simulink model "simulinkMonkey"  (R2019b)
settings: Solver=VariableStepAuto  StartTime=0.0  StopTime=3  RelTol=1e-3
values from neighbouring files (symbols this model uses):
  dq0_sim = T(1, 13:19)    [prepSimulink.m]
  q0_sim = T(1, 6:12)    [prepSimulink.m]
libraries: simulink x2
settings Model: Creator=Mike Dermksian  LastModifiedBy=Mike Dermksian

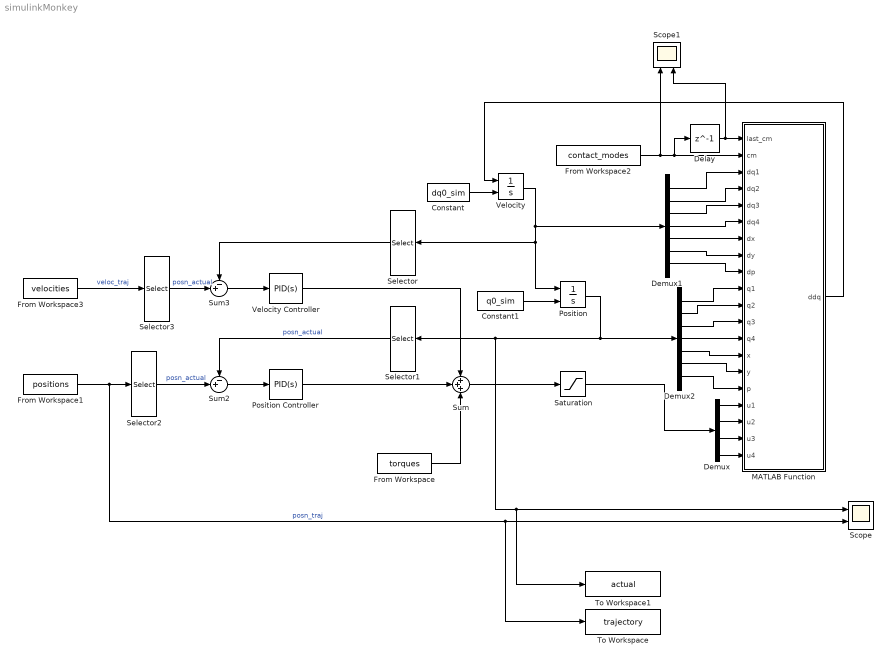
== system simulinkMonkey ==
  Constant : Constant  Value=dq0_sim
  Constant1 : Constant  Value=q0_sim
  Delay : Delay  DelayLength=1  InitialCondition=12
  Demux : Demux
  Demux1 : Demux  Outputs=7
  Demux2 : Demux  Outputs=7
  From Workspace : FromWorkspace  VariableName=torques  SampleTime=0  Interpolate=off  OutputAfterFinalValue=Setting to zero
  From Workspace1 : FromWorkspace  VariableName=positions  SampleTime=0  OutputAfterFinalValue=Holding final value
  From Workspace2 : FromWorkspace  VariableName=contact_modes  SampleTime=0  Interpolate=off  OutputAfterFinalValue=Holding final value
  From Workspace3 : FromWorkspace  VariableName=velocities  SampleTime=0  OutputAfterFinalValue=Holding final value
  MATLAB Function : MATLAB Function  TreatAsAtomicUnit=on
  Position : Integrator  InitialConditionSource=external
  Position Controller : simulink/Continuous/PID Controller  Controller=PID  Form=Parallel  TimeDomain=Continuous-time  SampleTime=-1  IntegratorMethod=Forward Euler  FilterMethod=Forward Euler  ControllerParametersSource=internal  P=100  I=10  D=0.1  UseFilter=on  N=100  TunerSelectOption=Transfer Function Based (PID Tuner App)  InitialConditionSource=internal  InitialConditionForIntegrator=0  InitialConditionForFilter=0  DifferentiatorICPrevScaledInput=0  ExternalReset=none  TrackingMode=off  Kt=1  LimitOutput=off  UpperSaturationLimit=inf  LowerSaturationLimit=-inf  LinearizeAsGain=on  AntiWindupMode=none  Kb=1  POutMin=[]  POutMax=[]  IOutMin=[]  IOutMax=[]  DOutMin=[]  DOutMax=[]  NOutMin=[]  NOutMax=[]  SumOutMin=[]  SumOutMax=[]  SaturationOutMin=[]  SaturationOutMax=[]  PParamMin=[]  PParamMax=[]  IParamMin=[]  IParamMax=[]  DParamMin=[]  DParamMax=[]  NParamMin=[]  NParamMax=[]  KbParamMin=[]  KbParamMax=[]  KtParamMin=[]  KtParamMax=[]  KbOutMin=[]  KbOutMax=[]  KtOutMin=[]  KtOutMax=[]  IntegratorOutMin=[]  IntegratorOutMax=[]  FilterOutMin=[]  FilterOutMax=[]  SumI1OutMin=[]  SumI1OutMax=[]  SumI2OutMin=[]  SumI2OutMax=[]  SumI3OutMin=[]  SumI3OutMax=[]  SumI4OutMin=[]  SumI4OutMax=[]  SumDOutMin=[]  SumDOutMax=[]  DifferentiatorOutMin=[]  DifferentiatorOutMax=[]  FilterDiffOutCoefMin=[]  FilterDiffOutCoefMax=[]  ReciprocalOutMin=[]  ReciprocalOutMax=[]  SumDenOutMin=[]  SumDenOutMax=[]  SumNumOutMin=[]  SumNumOutMax=[]  DivideOutMin=[]  DivideOutMax=[]  IntegratorContinuousStateAttributes=''  IntegratorStateMustResolveToSignalObject=off  IntegratorRTWStateStorageClass=Auto  FilterContinuousStateAttributes=''  FilterStateMustResolveToSignalObject=off  FilterRTWStateStorageClass=Auto  ParallelPVariant=InternalParameters  IdealPVariant=Disabled  IVariant=InternalParameters  DVariant=InternalParameters  IntegratorVariant=Continuous  SatVariant=Disabled  AWVariant=Passthrough  PCopyVariant=Disabled  TRVariant=Disabled  FdbkBlocksVariant=Forward  IdealPFdbkVariant=Disabled  SatFdbkVariant=Disabled  DerivativeFilterVariant=ContFilter  NVariant=InternalParameters  NCopyVariant=Disabled  FilterICVariant=InternalICsFilter  IntegratorICVariant=InternalICs  ExternalResetVariant=Disabled  TRSumVariant=Passthrough  SumFdbkVariant=Disabled  SumVariant=Sum_PID
  Saturation : Saturate  UpperLimit=3  LowerLimit=-3
  Scope : Scope  NumInputPorts=2
  Scope1 : Scope  NumInputPorts=2
  Selector{,1..3} (4 alike) : Selector  InputPortWidth=7  IndexOptions=Index vector (dialog)  Indices=[1 2 3 4]  OutputSizes=1
  Sum : Sum  Inputs=+++
  Sum2 : Sum  Inputs=-+|
  Sum3 : Sum  Inputs=-+|
  To Workspace : ToWorkspace  VariableName=trajectory  SampleTime=-1
  To Workspace1 : ToWorkspace  VariableName=actual  SampleTime=-1
  Velocity : Integrator  InitialConditionSource=external
  Velocity Controller : simulink/Continuous/PID Controller  Controller=PID  Form=Parallel  TimeDomain=Continuous-time  SampleTime=-1  IntegratorMethod=Forward Euler  FilterMethod=Forward Euler  ControllerParametersSource=internal  P=100  I=10  D=0.1  UseFilter=on  N=100  TunerSelectOption=Transfer Function Based (PID Tuner App)  InitialConditionSource=internal  InitialConditionForIntegrator=0  InitialConditionForFilter=0  DifferentiatorICPrevScaledInput=0  ExternalReset=none  TrackingMode=off  Kt=1  LimitOutput=off  UpperSaturationLimit=inf  LowerSaturationLimit=-inf  LinearizeAsGain=on  AntiWindupMode=none  Kb=1  POutMin=[]  POutMax=[]  IOutMin=[]  IOutMax=[]  DOutMin=[]  DOutMax=[]  NOutMin=[]  NOutMax=[]  SumOutMin=[]  SumOutMax=[]  SaturationOutMin=[]  SaturationOutMax=[]  PParamMin=[]  PParamMax=[]  IParamMin=[]  IParamMax=[]  DParamMin=[]  DParamMax=[]  NParamMin=[]  NParamMax=[]  KbParamMin=[]  KbParamMax=[]  KtParamMin=[]  KtParamMax=[]  KbOutMin=[]  KbOutMax=[]  KtOutMin=[]  KtOutMax=[]  IntegratorOutMin=[]  IntegratorOutMax=[]  FilterOutMin=[]  FilterOutMax=[]  SumI1OutMin=[]  SumI1OutMax=[]  SumI2OutMin=[]  SumI2OutMax=[]  SumI3OutMin=[]  SumI3OutMax=[]  SumI4OutMin=[]  SumI4OutMax=[]  SumDOutMin=[]  SumDOutMax=[]  DifferentiatorOutMin=[]  DifferentiatorOutMax=[]  FilterDiffOutCoefMin=[]  FilterDiffOutCoefMax=[]  ReciprocalOutMin=[]  ReciprocalOutMax=[]  SumDenOutMin=[]  SumDenOutMax=[]  SumNumOutMin=[]  SumNumOutMax=[]  DivideOutMin=[]  DivideOutMax=[]  IntegratorContinuousStateAttributes=''  IntegratorStateMustResolveToSignalObject=off  IntegratorRTWStateStorageClass=Auto  FilterContinuousStateAttributes=''  FilterStateMustResolveToSignalObject=off  FilterRTWStateStorageClass=Auto  ParallelPVariant=InternalParameters  IdealPVariant=Disabled  IVariant=InternalParameters  DVariant=InternalParameters  IntegratorVariant=Continuous  SatVariant=Disabled  AWVariant=Passthrough  PCopyVariant=Disabled  TRVariant=Disabled  FdbkBlocksVariant=Forward  IdealPFdbkVariant=Disabled  SatFdbkVariant=Disabled  DerivativeFilterVariant=ContFilter  NVariant=InternalParameters  NCopyVariant=Disabled  FilterICVariant=InternalICsFilter  IntegratorICVariant=InternalICs  ExternalResetVariant=Disabled  TRSumVariant=Passthrough  SumFdbkVariant=Disabled  SumVariant=Sum_PID
  wires:
  Velocity/1 -> Position/1, Selector/1, Demux1/1
  MATLAB Function/1(ddq) -> Velocity/1
  Position/1 -> Demux2/1, Scope/1, To Workspace1/1, Selector1/1
  Demux/1 -> MATLAB Function/17(u1)
  Demux/2 -> MATLAB Function/18(u2)
  Demux/3 -> MATLAB Function/19(u3)
  Demux/4 -> MATLAB Function/20(u4)
  Constant/1 -> Velocity/2
  Constant1/1 -> Position/2
  Sum/1 -> Saturation/1
  Sum2/1 -> Position Controller/1
  From Workspace1/1 -> To Workspace/1, Scope/2, Selector2/1  "posn_traj"
  From Workspace2/1 -> MATLAB Function/2(cm), Delay/1, Scope1/1
  Selector/1 -> Sum3/1
  Selector1/1 -> Sum2/1  "posn_actual"
  From Workspace3/1 -> Selector3/1  "veloc_traj"
  Sum3/1 -> Velocity Controller/1
  From Workspace/1 -> Sum/3
  Position Controller/1 -> Sum/2
  Velocity Controller/1 -> Sum/1
  Selector2/1 -> Sum2/2  "posn_actual"
  Selector3/1 -> Sum3/2  "posn_actual"
  Saturation/1 -> Demux/1
  Delay/1 -> Scope1/2, MATLAB Function/1(last_cm)
  Demux1/1 -> MATLAB Function/3(dq1)
  Demux1/2 -> MATLAB Function/4(dq2)
  Demux1/3 -> MATLAB Function/5(dq3)
  Demux1/4 -> MATLAB Function/6(dq4)
  Demux1/5 -> MATLAB Function/7(dx)
  Demux1/6 -> MATLAB Function/8(dy)
  Demux1/7 -> MATLAB Function/9(dp)
  Demux2/1 -> MATLAB Function/10(q1)
  Demux2/2 -> MATLAB Function/11(q2)
  Demux2/3 -> MATLAB Function/12(q3)
  Demux2/4 -> MATLAB Function/13(q4)
  Demux2/5 -> MATLAB Function/14(x)
  Demux2/6 -> MATLAB Function/15(y)
  Demux2/7 -> MATLAB Function/16(p)

== matlab function simulinkMonkey/MATLAB Function ==
  data: last_cm input; cm input; dq1 input; dq2 input; dq3 input; dq4 input; dx input; dy input; dp input; q1 input; q2 input; q3 input; q4 input; x input; y input; p input; ddq output; u1 input; u2 input; u3 input; u4 input
function ddq = fcn(last_cm,cm,dq1,dq2,dq3,dq4,dx,dy,dp,q1,q2,q3,q4,x,y,p,u1,u2,u3,u4)
q = [q1;q2;q3;q4;x;y;p];
dq = [dq1;dq2;dq3;dq4;dx;dy;dp];
if last_cm ~= cm
    switch cm
        case 1
            dq = dq - simulinkAdag1(q(7),q(1),q(2),q(3),q(4))'*simulinkA1(q(7),q(1),q(2))*dq;
        case 2
            dq = dq - simulinkAdag2(q(7),q(1),q(2),q(3),q(4))'*simulinkA2(q(7),q(3),q(4))*dq;
        case 12
            dq = dq - simulinkAdag12(q(7),q(1),q(2),q(3),q(4))'*simulinkA12(q(7),q(1),q(2),q(3),q(4))*dq;
        otherwise
            dq = zeros(7,1);
    end
end
switch cm
    case 1
        ddq = simulinkDynamics1(dq(7),dq(1),dq(2),dq(3),dq(4),q(7),q(1),q(2),q(3),q(4),u1,u2,u3,u4);
    case 2
        ddq = simulinkDynamics2(dq(7),dq(1),dq(2),dq(3),dq(4),q(7),q(1),q(2),q(3),q(4),u1,u2,u3,u4);
    case 12
        ddq = simulinkDynamics12(dq(7),dq(1),dq(2),dq(3),dq(4),q(7),q(1),q(2),q(3),q(4),u1,u2,u3,u4);
    otherwise
        ddq = zeros(7,1);
end
end
